simulink model "cpm_jap_r2019a"  (R2019a)
settings: Solver=ode4  StartTime=0.0  StopTime=inf  FixedStep=StepSize  RelTol=1e-3  EnableMultiTasking=on
PostLoadFcn:
  | %% PARAMETER INITIALIZATION
  | modelname = gcs;
  | p = Simulink.Mask.get([modelname, '/CP Model']);
  | 
  | %% HEART
  | % Basal heart period, T0 (s):
  | p.Parameters(1,1).Value = '0.58';
  | %% Right atrium
  | % RA Compliance, Cra (ml/mmHg):
  | p.Parameters(1,2).Value = '31.25';
  | % RA Resistance, Rra (mmHg s/ml):
  | p.Parameters(1,3).Value = '0.0025';
  | % RA Unstressed volume, Vu_ra (ml):
  | p.Parameters(1,4).Value = '22';
  | %% Left atrium
  | % LA Compliance, Cla (ml/mmHg):
  | p.Parameters(1,5).Value = '19.23';
  | % LA Resistance, Rla (mmHg s/ml):
  | p.Parameters(1,6).Value = '0.0025';
  | % LA Unstressed volume, Vu_la (ml):
  | p.Parameters(1,7).Value = '22';
  | %% Right ventricle
  | % RV Resistance coefficient, kR_rv (s/ml):
  | p.Parameters(1,8).Value = '0.0014';
  | % RV free wall End-systolic maximal elastance, Emax_rvf0 (mmHg/ml):
  | p.Parameters(1,9).Value = '1.412';
  | % RV free wall End-systolic unstressed volume, Vu_rvf (ml):
  | p.Parameters(1,10).Value = '35.904';
  | % RV free wall End-diastolic pressure intercept, P0_rvf (mmHg):
  | p.Parameters(1,11).Value = '1.5';
  | % RV free wall End-diastolic elastance coefficient, kE_rvf (1/ml):
  | p.Parameters(1,12).Value = '0.011';
  | % RV free wall Contraction delay (s):
  | p.Parameters(1,13).Value = '0';
  | %% Left ventricle
  | % LV Resistance coefficient, kR_lv (s/ml):
  | p.Parameters(1,14).Value = '0.00037';
  | % LV free wall End-systolic maximal elastance, Emax_lvf0 (mmHg/ml):
  | p.Parameters(1,15).Value = '2.392';
  | % LV free wall End-systolic unstressed volume, Vu_lvf (ml):
  | p.Parameters(1,16).Value = '14.7576';
  | % LV free wall End-diastolic pressure intercept, P0_lvf (mmHg):
  | p.Parameters(1,17).Value = '1.5';
  | % LV free wall End-diastolic elastance coefficient, kE_lvf (1/ml):
  | p.Parameters(1,18).Value = '0.014';
  | % LV Contraction delay (s):
  | p.Parameters(1,19).Value = '0';
  | %% Septum
  | % Septal End-systolic maximal elastance, Emax_spt0 (mmHg/ml):
  | p.Parameters(1,20).Value = '32.4';
  | % Septal End-systolic unstressed volume, Vu_spt (ml):
  | p.Parameters(1,21).Value = '0';
  | % Septal End-diastolic pressure intercept, P0_spt (mmHg):
  | p.Parameters(1,22).Value = '1.11';
  | % Septal End-diastolic elastance coefficient, kE_spt (1/ml):
  | p.Parameters(1,23).Value = '0.175';
  | %% Pericardium
  | % Pericardial Unstressed volume, Vu_pcd (ml):
  | p.Parameters(1,24).Value = '200';
  | % Pericardial Pressure intercept, P0_pcd (mmHg):
  | p.Parameters(1,25).Value = '0.5';
  | % Pericardial Elastance coefficient, kE_pcd (1/ml):
  | p.Parameters(1,26).Value = '0.005';
  | % Pericardial volume, V_pcd (ml):
  | p.Parameters(1,27).Value = '40';
  | 
  | %% LUNGS
  | % Endotracheal tube resistance, Ret (cmH2O/l/s):
  | p.Parameters(1,28).Value = '0';
  | % Lungs resistance, R_L (cmH2O/l/s):
  | p.Parameters(1,29).Value = '1.7459';
  | % Lungs compliance, C_L (l/cmH2O):
  | p.Parameters(1,30).Value = '0.2';
  | % Lungs unstressed volume, Vu_L (l):
  | p.Parameters(1,31).Value = '1.25';
  | % Chest wall compliance, C_cw (l/cmH2O):
  | p.Parameters(1,32).Value = '0.2445';
  | % Chest wall unstressed volume, Vu_cw (l):
  | p.Parameters(1,33).Value = '3.473';
  | % Basal amplitude (cmH2O):
  | p.Parameters(1,34).Value = '5';
  | % Basal frequency (breaths/min):
  | p.Parameters(1,35).Value = '12';
  | % I:E ratio:
  | p.Parameters(1,36).Value = '0.6';
  | % Check for passive patient:
  | p.Parameters(1,37).Value = 'off';
  | % Change in expiratory resistance value (for COPD cases):
  | p.Parameters(1,38).Value = '1';
  | 
  | %% CIRCULATION
  | %% Systemic arteries
  | % Systemic arterial Compliance, Csa (ml/mmHg):
  | p.Parameters(1,39).Value = '0.28';
  | % Systemic arterial Resistance, Rsa (mmHg s/ml):
  | p.Parameters(1,40).Value = '0.06';
  | % Systemic arterial Inertance, Lsa (mmHg ml/s^2):
  | p.Parameters(1,41).Value = '0.00022';
  | % Systemic arterial Unstressed volume, Vu_sa (ml):
  | p.Parameters(1,42).Value = '0';
  | %% Systemic Splanchnic
  | % Systemic Splanchnic peripheral Compliance, Csp (ml/mmHg):
  | p.Parameters(1,43).Value = '2.05';
  | % Systemic Splanchnic peripheral Basal resistance, Rsp_0 (mmHg s/ml):
  | p.Parameters(1,44).Value = '2.49';
  | % Systemic Splanchnic peripheral Unstressed volume, Vu_sp (ml):
  | p.Parameters(1,45).Value = '274.4';
  | % Systemic Splanchnic venous Compliance, Csv (ml/mmHg):
  | p.Parameters(1,46).Value = '42.777';
  | % Systemic Splanchnic venous Resistance, Rsv (mmHg s/ml):
  | p.Parameters(1,47).Value = '0.038';
  | % Systemic Splanchnic venous Basal unstressed volume, Vu_sv_0 (ml):
  | p.Parameters(1,48).Value = '1435.4';
  | %% Systemic Extrasplanchnic
  | % Systemic Extrasplanchnic peripheral Compliance, Cep (ml/mmHg):
  | p.Parameters(1,49).Value = '1.67';
  | % Systemic Extrasplanchnic peripheral Basal resistance, Rep_0 (mmHg s/ml):
  | p.Parameters(1,50).Value = '0.78';
  | % Systemic Extrasplanchnic peripheral Unstressed volume, Vu_ep (ml):
  | p.Parameters(1,51).Value = '336.6';
  | % Systemic Extrasplanchnic venous Compliance, Cev (ml/mmHg):
  | p.Parameters(1,52).Value = '35';
  | % Systemic Extrasplanchnic venous Resistance, Rev (mmHg s/ml):
  | p.Parameters(1,53).Value = '0.016';
  | % Systemic Extrasplanchnic venous Basal unstressed volume, Vu_ev_0 (ml):
  | p.Parameters(1,54).Value = '1537';
  | %% Thoracic veins
  | % Thoracic veins Compliance, Cvc (ml/mmHg):
  | p.Parameters(1,55).Value = '6.6667';
  | % Thoracic veins Basal resistance, Rvc_0 (mmHg s/ml):
  | p.Parameters(1,56).Value = '0.025';
  | % Thoracic veins Unstressed volume, Vu_vc (ml):
  | p.Parameters(1,57).Value = '130';
  | %% Pulmonary arteries
  | % Pulmonary arterial Compliance, Cpa (ml/mmHg):
  | p.Parameters(1,58).Value = '0.76';
  | % Pulmonary arterial Resistance, Rpa (mmHg s/ml):
  | p.Parameters(1,59).Value = '0.023';
  | % Pulmonary arterial Inertance, Lpa (mmHg ml/s^2):
  | p.Parameters(1,60).Value = '0.00018';
  | % Pulmonary arterial Unstressed volume, Vu_pa (ml):
  | p.Parameters(1,61).Value = '0';
  | %% Pulmonary peripheral vessels
  | % Pulmonary peripheral Compliance, Cpp_tot (ml/mmHg):
  | p.Parameters(1,62).Value = '5.80';
  | % Pulmonary peripheral Resistance, Rpp_tot (mmHg s/ml):
  | p.Parameters(1,63).Value = '0.0894';
  | % Pulmonary peripheral Unstressed volume, Vu_pp (ml):
  | p.Parameters(1,64).Value = '108.24';
  | %% Pulmonary veins
  | % Pulmonary venous Compliance, Cpv (ml/mmHg):
  | p.Parameters(1,65).Value = '25.37';
  | % Pulmonary venous Resistance, Rpv (mmHg s/ml):
  | p.Parameters(1,66).Value = '0.0056';
  | % Pulmonary venous Unstressed volume, Vu_pv (ml):
  | p.Parameters(1,67).Value = '105.6';
  | % Basal blood volume, Vt (ml):
  | p.Parameters(1,68).Value = '5300';
  | % Blood infusion Enable?
  | p.Parameters(1,69).Value = 'off';
  | % Blood infusion Duration (min):
  | p.Parameters(1,70).Value = '30';
  | % Blood infusion Volume (ml):
  | p.Parameters(1,71).Value = '500';
  | 
  | %% NEURAL
  | %% Receptors
  | % Baroreceptors set point (mmHg):
  | p.Parameters(1,72).Value = '92';
  | % Baroreceptors Sensitivity (mmHg):
  | p.Parameters(1,73).Value = '11.758';
  | % Central chemoreceptors set point (mmHg):
  | p.Parameters(1,74).Value = '40';
  | % Peripheral chemoreceptors set point (spike/s):
  | p.Parameters(1,75).Value = '3.60';
  | % Central chemoreceptors ampl. sensitivity (dyn/cm^2/mmHg):
  | p.Parameters(1,76).Value = '850';
  | % Perip. chemoreceptors ampl. sensitivity (dyn/cm^2/sp/s):
  | p.Parameters(1,77).Value = '1310';
  | % Central chemoreceptors freq. sensitivity (bpm/mmHg):
  | p.Parameters(1,78).Value = '0.9';
  | % Perip. chemoreceptors freq. sensitivity (bpm/sp/s):
  | p.Parameters(1,79).Value = '0.873474';
  | % Lung-stretch receptors Sensitivity (spkes/l/s)
  | p.Parameters(1,80).Value = '11.76';
  | %% Sympathetic
  | % Baroreceptors's sympathetic influence on heart
  | p.Parameters(1,81).Value = '-1.75';
  | % Peripheral chemoreceptors's sympathetic influence on heart
  | p.Parameters(1,82).Value = '1';
  | % Lung-stretch receptors's sympathetic influence on heart
  | p.Parameters(1,83).Value = '0';
  | % Baroreceptors's sympathetic influence on peripheral circulation
  | p.Parameters(1,84).Value = '-1.1375';
  | % Peripheral chemoreceptors's sympathetic influence on peripheral circulation
  | p.Parameters(1,85).Value = '1.716';
  | % Lung-stretch receptors's sympathetic influence on peripheral circulation
  | p.Parameters(1,86).Value = '-0.3997';
  | % Baroreceptors's sympathetic influence on venous circulation
  | p.Parameters(1,87).Value = '-1.0806';
  | % Peripheral chemoreceptors's sympathetic influence on venous circulation
  | p.Parameters(1,88).Value = '1.716';
  | % Lung-stretch receptors's sympathetic influence on venous circulation
  | p.Parameters(1,89).Value = '-0.2907';
  | %% Vagal
  | % Baroreceptors's vagal influence on heart
  | p.Parameters(1,90).Value = '7.06';
  | % Peripheral chemoreceptors's vagal influence on peripheral circulation
  | p.Parameters(1,91).Value = '0.208';
  | % Peripheral chemoreceptors's vagal influence on venous circulation
  | p.Parameters(1,92).Value = '-0.103';
  | %% CNS Ischemic response
  | % PO2 sensitivity heart (mmHg):
  | p.Parameters(1,93).Value = '45';
  | % PO2 sensitivity peripheral circulation (mmHg):
  | p.Parameters(1,94).Value = '30';
  | % PO2 sensitivity venous circulation (mmHg):
  | p.Parameters(1,95).Value = '30';
  | % PCO2 sensitivity heart (1/(mmHg s)):
  | p.Parameters(1,96).Value = '1';
  | % PCO2 sensitivity peripheral circulation (1/(mmHg s)):
  | p.Parameters(1,97).Value = '1.5';
  | % PCO2 sensitivity Veins (1/(mmHg s)):
  | p.Parameters(1,98).Value = '0';
  | 
  | %% METABOLISM
  | % Splanchnic Oxygen consumption (ml/min):
  | p.Parameters(1,99).Value = '108.419';
  | % Splanchnic Carbon dioxide production (ml/min):
  | p.Parameters(1,100).Value = '91.072';
  | % Splanchnic Tissue volume (ml):
  | p.Parameters(1,101).Value = '2673';
  | % Extrasplanchnic Oxygen consumption (ml/min):
  | p.Parameters(1,102).Value = '137.785';
  | % Extrasplanchnic Carbon dioxide production (ml/min):
  | p.Parameters(1,103).Value = '115.7394';
  | % Extrasplanchnic Tissue volume (ml):
  | p.Parameters(1,104).Value = '33046';
  | 
  | %% GAS EXCHANGE
  | % Oxygen air fraction, FiO2 (%):
  | p.Parameters(1,105).Value = '21.0379';
  | % Carbon dioxide air fraction, FiCO2 (%):
  | p.Parameters(1,106).Value = '0.042076';
  | % Pulmonary shunt, sh (%):
  | p.Parameters(1,107).Value = '1.7';
  | % Deadspace volume, Vdead (l):
  | p.Parameters(1,108).Value = '0.15';
InitFcn:
  | logFreq = 100; % logging frequency
  | StepSize = 5e-4; % simulation step size
  | 
  | %% PARAMETER INITIALIZATION
  | modelname = gcs;
  | p = Simulink.Mask.get([modelname, '/CP Model']);
  | 
  | %% HEART
  | % Basal heart period, T0 (s):
  | p.Parameters(1,1).Value = '0.58';
  | %% Right atrium
  | % RA Compliance, Cra (ml/mmHg):
  | p.Parameters(1,2).Value = '31.25';
  | % RA Resistance, Rra (mmHg s/ml):
  | p.Parameters(1,3).Value = '0.0025';
  | % RA Unstressed volume, Vu_ra (ml):
  | p.Parameters(1,4).Value = '22';
  | %% Left atrium
  | % LA Compliance, Cla (ml/mmHg):
  | p.Parameters(1,5).Value = '19.23';
  | % LA Resistance, Rla (mmHg s/ml):
  | p.Parameters(1,6).Value = '0.0025';
  | % LA Unstressed volume, Vu_la (ml):
  | p.Parameters(1,7).Value = '22';
  | %% Right ventricle
  | % RV Resistance coefficient, kR_rv (s/ml):
  | p.Parameters(1,8).Value = '0.0014';
  | % RV free wall End-systolic maximal elastance, Emax_rvf0 (mmHg/ml):
  | p.Parameters(1,9).Value = '1.412';
  | % RV free wall End-systolic unstressed volume, Vu_rvf (ml):
  | p.Parameters(1,10).Value = '35.904';
  | % RV free wall End-diastolic pressure intercept, P0_rvf (mmHg):
  | p.Parameters(1,11).Value = '1.5';
  | % RV free wall End-diastolic elastance coefficient, kE_rvf (1/ml):
  | p.Parameters(1,12).Value = '0.011';
  | % RV free wall Contraction delay (s):
  | p.Parameters(1,13).Value = '0';
  | %% Left ventricle
  | % LV Resistance coefficient, kR_lv (s/ml):
  | p.Parameters(1,14).Value = '0.00037';
  | % LV free wall End-systolic maximal elastance, Emax_lvf0 (mmHg/ml):
  | p.Parameters(1,15).Value = '2.392';
  | % LV free wall End-systolic unstressed volume, Vu_lvf (ml):
  | p.Parameters(1,16).Value = '14.7576';
  | % LV free wall End-diastolic pressure intercept, P0_lvf (mmHg):
  | p.Parameters(1,17).Value = '1.5';
  | % LV free wall End-diastolic elastance coefficient, kE_lvf (1/ml):
  | p.Parameters(1,18).Value = '0.014';
  | % LV Contraction delay (s):
  | p.Parameters(1,19).Value = '0';
  | %% Septum
  | % Septal End-systolic maximal elastance, Emax_spt0 (mmHg/ml):
  | p.Parameters(1,20).Value = '32.4';
  | % Septal End-systolic unstressed volume, Vu_spt (ml):
  | p.Parameters(1,21).Value = '0';
  | % Septal End-diastolic pressure intercept, P0_spt (mmHg):
  | p.Parameters(1,22).Value = '1.11';
  | % Septal End-diastolic elastance coefficient, kE_spt (1/ml):
  | p.Parameters(1,23).Value = '0.175';
  | %% Pericardium
  | % Pericardial Unstressed volume, Vu_pcd (ml):
  | p.Parameters(1,24).Value = '200';
  | % Pericardial Pressure intercept, P0_pcd (mmHg):
  | p.Parameters(1,25).Value = '0.5';
  | % Pericardial Elastance coefficient, kE_pcd (1/ml):
  | p.Parameters(1,26).Value = '0.005';
  | % Pericardial volume, V_pcd (ml):
  | p.Parameters(1,27).Value = '40';
  | 
  | %% LUNGS
  | % Endotracheal tube resistance, Ret (cmH2O/l/s):
  | p.Parameters(1,28).Value = '0';
  | % Lungs resistance, R_L (cmH2O/l/s):
  | p.Parameters(1,29).Value = '1.7459';
  | % Lungs compliance, C_L (l/cmH2O):
  | p.Parameters(1,30).Value = '0.2';
  | % Lungs unstressed volume, Vu_L (l):
  | p.Parameters(1,31).Value = '1.25';
  | % Chest wall compliance, C_cw (l/cmH2O):
  | p.Parameters(1,32).Value = '0.2445';
  | % Chest wall unstressed volume, Vu_cw (l):
  | p.Parameters(1,33).Value = '3.473';
  | % Basal amplitude (cmH2O):
  | p.Parameters(1,34).Value = '5';
  | % Basal frequency (breaths/min):
  | p.Parameters(1,35).Value = '12';
  | % I:E ratio:
  | p.Parameters(1,36).Value = '0.6';
  | % Check for passive patient:
  | p.Parameters(1,37).Value = 'off';
  | % Change in expiratory resistance value (for COPD cases):
  | p.Parameters(1,38).Value = '1';
  | 
  | %% CIRCULATION
  | %% Systemic arteries
  | % Systemic arterial Compliance, Csa (ml/mmHg):
  | p.Parameters(1,39).Value = '0.28';
  | % Systemic arterial Resistance, Rsa (mmHg s/ml):
  | p.Parameters(1,40).Value = '0.06';
  | % Systemic arterial Inertance, Lsa (mmHg ml/s^2):
  | p.Parameters(1,41).Value = '0.00022';
  | % Systemic arterial Unstressed volume, Vu_sa (ml):
  | p.Parameters(1,42).Value = '0';
  | %% Systemic Splanchnic
  | % Systemic Splanchnic peripheral Compliance, Csp (ml/mmHg):
  | p.Parameters(1,43).Value = '2.05';
  | % Systemic Splanchnic peripheral Basal resistance, Rsp_0 (mmHg s/ml):
  | p.Parameters(1,44).Value = '2.49';
  | % Systemic Splanchnic peripheral Unstressed volume, Vu_sp (ml):
  | p.Parameters(1,45).Value = '274.4';
  | % Systemic Splanchnic venous Compliance, Csv (ml/mmHg):
  | p.Parameters(1,46).Value = '42.777';
  | % Systemic Splanchnic venous Resistance, Rsv (mmHg s/ml):
  | p.Parameters(1,47).Value = '0.038';
  | % Systemic Splanchnic venous Basal unstressed volume, Vu_sv_0 (ml):
  | p.Parameters(1,48).Value = '1435.4';
  | %% Systemic Extrasplanchnic
  | % Systemic Extrasplanchnic peripheral Compliance, Cep (ml/mmHg):
  | p.Parameters(1,49).Value = '1.67';
  | % Systemic Extrasplanchnic peripheral Basal resistance, Rep_0 (mmHg s/ml):
  | p.Parameters(1,50).Value = '0.78';
  | % Systemic Extrasplanchnic peripheral Unstressed volume, Vu_ep (ml):
  | p.Parameters(1,51).Value = '336.6';
  | % Systemic Extrasplanchnic venous Compliance, Cev (ml/mmHg):
  | p.Parameters(1,52).Value = '35';
  | % Systemic Extrasplanchnic venous Resistance, Rev (mmHg s/ml):
  | p.Parameters(1,53).Value = '0.016';
  | % Systemic Extrasplanchnic venous Basal unstressed volume, Vu_ev_0 (ml):
  | p.Parameters(1,54).Value = '1537';
  | %% Thoracic veins
  | % Thoracic veins Compliance, Cvc (ml/mmHg):
  | p.Parameters(1,55).Value = '6.6667';
  | % Thoracic veins Basal resistance, Rvc_0 (mmHg s/ml):
  | p.Parameters(1,56).Value = '0.025';
  | % Thoracic veins Unstressed volume, Vu_vc (ml):
  | p.Parameters(1,57).Value = '130';
  | %% Pulmonary arteries
  | % Pulmonary arterial Compliance, Cpa (ml/mmHg):
  | p.Parameters(1,58).Value = '0.76';
  | % Pulmonary arterial Resistance, Rpa (mmHg s/ml):
  | p.Parameters(1,59).Value = '0.023';
  | % Pulmonary arterial Inertance, Lpa (mmHg ml/s^2):
  | p.Parameters(1,60).Value = '0.00018';
  | % Pulmonary arterial Unstressed volume, Vu_pa (ml):
  | p.Parameters(1,61).Value = '0';
  | %% Pulmonary peripheral vessels
  | % Pulmonary peripheral Compliance, Cpp_tot (ml/mmHg):
  | p.Parameters(1,62).Value = '5.80';
  | % Pulmonary peripheral Resistance, Rpp_tot (mmHg s/ml):
  | p.Parameters(1,63).Value = '0.0894';
  | % Pulmonary peripheral Unstressed volume, Vu_pp (ml):
  | p.Parameters(1,64).Value = '108.24';
  | %% Pulmonary veins
  | % Pulmonary venous Compliance, Cpv (ml/mmHg):
  | p.Parameters(1,65).Value = '25.37';
  | % Pulmonary venous Resistance, Rpv (mmHg s/ml):
  | p.Parameters(1,66).Value = '0.0056';
  | % Pulmonary venous Unstressed volume, Vu_pv (ml):
  | p.Parameters(1,67).Value = '105.6';
  | % Basal blood volume, Vt (ml):
  | p.Parameters(1,68).Value = '5300';
  | % Blood infusion Enable?
  | p.Parameters(1,69).Value = 'off';
  | % Blood infusion Duration (min):
  | p.Parameters(1,70).Value = '30';
  | % Blood infusion Volume (ml):
  | p.Parameters(1,71).Value = '500';
  | 
  | %% NEURAL
  | %% Receptors
  | % Baroreceptors set point (mmHg):
  | p.Parameters(1,72).Value = '92';
  | % Baroreceptors Sensitivity (mmHg):
  | p.Parameters(1,73).Value = '11.758';
  | % Central chemoreceptors set point (mmHg):
  | p.Parameters(1,74).Value = '40';
  | % Peripheral chemoreceptors set point (spike/s):
  | p.Parameters(1,75).Value = '3.60';
  | % Central chemoreceptors ampl. sensitivity (dyn/cm^2/mmHg):
  | p.Parameters(1,76).Value = '850';
  | % Perip. chemoreceptors ampl. sensitivity (dyn/cm^2/sp/s):
  | p.Parameters(1,77).Value = '1310';
  | % Central chemoreceptors freq. sensitivity (bpm/mmHg):
  | p.Parameters(1,78).Value = '0.9';
  | % Perip. chemoreceptors freq. sensitivity (bpm/sp/s):
  | p.Parameters(1,79).Value = '0.873474';
  | % Lung-stretch receptors Sensitivity (spkes/l/s)
  | p.Parameters(1,80).Value = '11.76';
  | %% Sympathetic
  | % Baroreceptors's sympathetic influence on heart
  | p.Parameters(1,81).Value = '-1.75';
  | % Peripheral chemoreceptors's sympathetic influence on heart
  | p.Parameters(1,82).Value = '1';
  | % Lung-stretch receptors's sympathetic influence on heart
  | p.Parameters(1,83).Value = '0';
  | % Baroreceptors's sympathetic influence on peripheral circulation
  | p.Parameters(1,84).Value = '-1.1375';
  | % Peripheral chemoreceptors's sympathetic influence on peripheral circulation
  | p.Parameters(1,85).Value = '1.716';
  | % Lung-stretch receptors's sympathetic influence on peripheral circulation
  | p.Parameters(1,86).Value = '-0.3997';
  | % Baroreceptors's sympathetic influence on venous circulation
  | p.Parameters(1,87).Value = '-1.0806';
  | % Peripheral chemoreceptors's sympathetic influence on venous circulation
  | p.Parameters(1,88).Value = '1.716';
  | % Lung-stretch receptors's sympathetic influence on venous circulation
  | p.Parameters(1,89).Value = '-0.2907';
  | %% Vagal
  | % Baroreceptors's vagal influence on heart
  | p.Parameters(1,90).Value = '7.06';
  | % Peripheral chemoreceptors's vagal influence on peripheral circulation
  | p.Parameters(1,91).Value = '0.208';
  | % Peripheral chemoreceptors's vagal influence on venous circulation
  | p.Parameters(1,92).Value = '-0.103';
  | %% CNS Ischemic response
  | % PO2 sensitivity heart (mmHg):
  | p.Parameters(1,93).Value = '45';
  | % PO2 sensitivity peripheral circulation (mmHg):
  | p.Parameters(1,94).Value = '30';
  | % PO2 sensitivity venous circulation (mmHg):
  | p.Parameters(1,95).Value = '30';
  | % PCO2 sensitivity heart (1/(mmHg s)):
  | p.Parameters(1,96).Value = '1';
  | % PCO2 sensitivity peripheral circulation (1/(mmHg s)):
  | p.Parameters(1,97).Value = '1.5';
  | % PCO2 sensitivity Veins (1/(mmHg s)):
  | p.Parameters(1,98).Value = '0';
  | 
  | %% METABOLISM
  | % Splanchnic Oxygen consumption (ml/min):
  | p.Parameters(1,99).Value = '108.419';
  | % Splanchnic Carbon dioxide production (ml/min):
  | p.Parameters(1,100).Value = '91.072';
  | % Splanchnic Tissue volume (ml):
  | p.Parameters(1,101).Value = '2673';
  | % Extrasplanchnic Oxygen consumption (ml/min):
  | p.Parameters(1,102).Value = '137.785';
  | % Extrasplanchnic Carbon dioxide production (ml/min):
  | p.Parameters(1,103).Value = '115.7394';
  | % Extrasplanchnic Tissue volume (ml):
  | p.Parameters(1,104).Value = '33046';
  | 
  | %% GAS EXCHANGE
  | % Oxygen air fraction, FiO2 (%):
  | p.Parameters(1,105).Value = '21.0379';
  | % Carbon dioxide air fraction, FiCO2 (%):
  | p.Parameters(1,106).Value = '0.042076';
  | % Pulmonary shunt, sh (%):
  | p.Parameters(1,107).Value = '1.7';
  | % Deadspace volume, Vdead (l):
  | p.Parameters(1,108).Value = '0.15';
StopFcn:
  | cpmResults = cpm_jap{1}.Values;
(part 1 of 2)
settings Model: ParamWorkspaceSource=ReferencedWorkspace  TunableVars=BreathAmp,BreathFreq,CL,C_cw,C_vc,Cep,Cev,Cla,ConsCO2Exspl,ConsCO2Spl,ConsO2Exspl,ConsO2Spl,Cpa,Cpp_tot,Cpv,Cra,Csa,Csp,Csv,Ees_spt0,Emax_lvf0,Emax_rvf0,ExsplVolume,FRCnom,FiCO2,FiO2,Gc_A_up,Gc_f_up,Gp_A_up,Gp_f_up,Gsr,IEratio,Lpa,Lsa,P0_lvf,P0_pcd,P0_rvf,P0_spt,PO2sh,PO2sp,PO2sv,PaCO2n,Pn,RL,R_vc_0,Rep_0,Ret,Rev,Rla,Rpa,Rpp_tot,Rpv,Rra,Rsa,Rsp_0,Rsv,SplVolume,T0,V0_pcd,V0_spt,V_pcd,Vdead,Vt,Vu_L,Vu_cw,Vu_ep,Vu_ev0,Vu_la,Vu_lvf,Vu_pa,Vu_pp,Vu_ps,Vu_pv,Vu_ra,Vu_rvf,Vu_sa,Vu_sp,Vu_sv0,Vu_vc,Wbsh,Wbsp,Wbsv,Wpcsh,Wpcsp,Wpcsv,Wpcv,Wsrsh,Wsrsp,Wsrsv,Wsrv,fapcn,gccsh,gccsp,gccsv,infusionDur,kBloodLoss,kE_lvf,kE_rvf,kRL_out,kR_lv,kR_rv,kab,kev,lambda_pcd,lambda_spt,lvContractionDelay,passivePatient,pumpFlag,rvContractionDelay,sh,volumeInfused  TunableVarsStorageClass=Auto,Auto,Auto,Auto,Auto,Auto,Auto,Auto,Auto,Auto,Auto,Auto,Auto,Auto,Auto,Auto,Auto,Auto,Auto,Auto,Auto,Auto,Auto,Auto,Auto,Auto,Auto,Auto,Auto,Auto,Auto,Auto,Auto,Auto,Auto,Auto,Auto,Auto,Auto,Auto,Auto,Auto,Auto,Auto,Auto,Auto,Auto,Auto,Auto,Auto,Auto,Auto,Auto,Auto,Auto,Auto,Auto,Auto,Auto,Auto,Auto,Auto,Auto,Auto,Auto,Auto,Auto,Auto,Auto,Auto,Auto,Auto,Auto,Auto,Auto,Auto,Auto,Auto,Auto,Auto,Auto,Auto,Auto,Auto,Auto,Auto,Auto,Auto,Auto,Auto,Auto,Auto,Auto,Auto,Auto,Auto,Auto,Auto,Auto,Auto,Auto,Auto,Auto,Auto,Auto,Auto,Auto,Auto,Auto,Auto,Auto  TunableVarsTypeQualifier=,,,,,,,,,,,,,,,,,,,,,,,,,,,,,,,,,,,,,,,,,,,,,,,,,,,,,,,,,,,,,,,,,,,,,,,,,,,,,,,,,,,,,,,,,,,,,,,,,,,,,,,,,,,,,,  Creator=nikolaos  LastModifiedBy=nikolaos
settings DataIOCC: SaveOutput=off  SaveTime=off  ReturnWorkspaceOutputs=off  SignalLoggingName=cpm_jap
settings OptimizationCC: BlockReduction=off  DefaultParameterBehavior=Inlined  OptimizeBlockIOStorage=off  BufferReuse=off  GlobalBufferReuse=off  ExpressionFolding=off  LocalBlockOutputs=off  OptimizeDataStoreBuffers=off  BusAssignmentInplaceUpdate=off
settings DebuggingCC: UnderspecifiedInitializationDetection=Classic  MergeDetectMultiDrivingBlocksExec=none  PregeneratedLibrarySubsystemCodeDiagnostic=none  ArithmeticOperatorsInVariantConditions=warning
settings SFSimCC: SimUseLocalCustomCode=off
settings RTWCC: RTWUseLocalCustomCode=off
settings ConfigComp: CovMetricSettings=dw  CovHtmlReporting=on  CovSaveCumulativeToWorkspaceVar=on  CovSaveSingleToWorkspaceVar=on  CovExternalEMLEnable=off

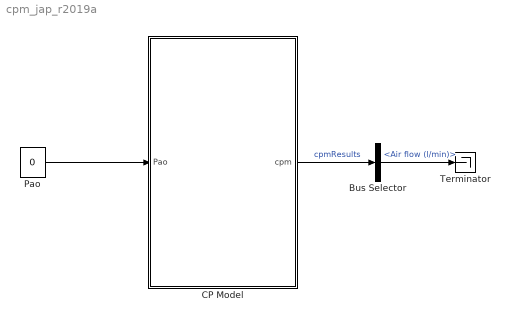
== system cpm_jap_r2019a ==
  Bus Selector : BusSelector  OutputSignals=lungs.Air flow (l/min)
  CP Model : Subsystem  mask(CP Model){sfcnParam58=0.58, sfcnParam16=31.25, sfcnParam53=0.0025, sfcnParam74=22, sfcnParam8=19.23, sfcnParam49=0.0025, sfcnParam68=22, sfcnParam101=0.0014, sfcnParam22=1.412, sfcnParam75=35.904, sfcnParam37=1.5, sfcnParam98=0.011, sfcnParam109=0, sfcnParam100=0.00037, sfcnParam21=2.392, sfcnParam69=14.7576, sfcnParam35=1.5, sfcnParam97=0.014, sfcnParam106=0, sfcnParam20=32.4, sfcnParam60=0, sfcnParam38=1.11, sfcnParam105=0.175, sfcnParam59=200, sfcnParam36=0.5, sfcnParam104=0.005, sfcnParam61=40, sfcnParam47=0, sfcnParam44=1.7459, sfcnParam3=0.2, sfcnParam64=1.25, sfcnParam4=0.2445, sfcnParam65=3.473, sfcnParam1=5, sfcnParam2=12, sfcnParam32=0.6, sfcnParam107=off, sfcnParam99=1, sfcnParam17=0.28, sfcnParam54=0.06, sfcnParam34=0.00022, sfcnParam76=0, sfcnParam18=2.05, sfcnParam55=2.49, sfcnParam77=274.4, sfcnParam19=42.777, sfcnParam56=0.038, sfcnParam78=1435.4, sfcnParam6=1.67, sfcnParam46=0.78, sfcnParam66=336.6, sfcnParam7=35, sfcnParam48=0.016, sfcnParam67=1537, sfcnParam5=6.6667, sfcnParam45=0.025, sfcnParam79=130, sfcnParam13=0.76, sfcnParam50=0.023, sfcnParam33=0.00018, sfcnParam70=0, sfcnParam14=5.80, sfcnParam51=0.0894, sfcnParam71=108.24, sfcnParam15=25.37, sfcnParam52=0.0056, sfcnParam73=105.6, sfcnParam63=5300, sfcnParam108=off, sfcnParam95=30, sfcnParam111=500, sfcnParam43=92, sfcnParam102=11.758, sfcnParam42=40, sfcnParam91=3.60, sfcnParam27=850, sfcnParam29=1310, sfcnParam28=0.9, sfcnParam30=0.873474, sfcnParam31=11.76, sfcnParam80=-1.75, sfcnParam83=1, sfcnParam87=0, sfcnParam81=-1.1375, sfcnParam84=1.716, sfcnParam88=-0.3997, sfcnParam82=-1.0806, sfcnParam85=1.716, sfcnParam89=-0.2907, sfcnParam103=7.06, sfcnParam86=0.208, sfcnParam90=-0.103, sfcnParam39=45, sfcnParam40=30, sfcnParam41=30, sfcnParam92=1, sfcnParam93=1.5, sfcnParam94=0, sfcnParam12=108.419, sfcnParam10=91.072, sfcnParam57=2673, sfcnParam11=137.785, sfcnParam9=115.7394, sfcnParam23=33046, sfcnParam26=21.0379, sfcnParam25=0.042076, sfcnParam110=1.7, sfcnParam62=0.15}
      mask prompts: sfcnParam58 "Basal heart period, T0 (s):"; sfcnParam16 "Compliance, Cra (ml/mmHg):"; sfcnParam53 "Resistance, Rra (mmHg s/ml):"; sfcnParam74 "Unstressed volume, Vu_ra (ml):"; sfcnParam8 "Compliance, Cla (ml/mmHg):"; sfcnParam49 "Resistance, Rla (mmHg s/ml):"; sfcnParam68 "Unstressed volume, Vu_la (ml):"; sfcnParam101 "Resistance coefficient, kR_rv (s/ml):"; sfcnParam22 "End-systolic maximal elastance, Emax_rvf0 (mmHg/ml):"; sfcnParam75 "End-systolic unstressed volume, Vu_rvf (ml):"; sfcnParam37 "End-diastolic pressure intercept, P0_rvf (mmHg):"; sfcnParam98 "End-diastolic elastance coefficient, kE_rvf (1/ml):"; sfcnParam109 "Contraction delay (s):"; sfcnParam100 "Resistance coefficient, kR_lv (s/ml):"; sfcnParam21 "End-systolic maximal elastance, Emax_lvf0 (mmHg/ml):"; sfcnParam69 "End-systolic unstressed volume, Vu_lvf (ml):"; sfcnParam35 "End-diastolic pressure intercept, P0_lvf (mmHg):"; sfcnParam97 "End-diastolic elastance coefficient, kE_lvf (1/ml):"; sfcnParam106 "Contraction delay (s):"; sfcnParam20 "End-systolic maximal elastance, Emax_spt0 (mmHg/ml):"; sfcnParam60 "End-systolic unstressed volume, Vu_spt (ml):"; sfcnParam38 "End-diastolic pressure intercept, P0_spt (mmHg):"; sfcnParam105 "End-diastolic elastance coefficient, kE_spt (1/ml):"; sfcnParam59 "Unstressed volume, Vu_pcd (ml):"; sfcnParam36 "Pressure intercept, P0_pcd (mmHg):"; sfcnParam104 "Elastance coefficient, kE_pcd (1/ml):"; sfcnParam61 "Pericardial volume, V_pcd (ml):"; sfcnParam47 "Endotracheal tube resistance, Ret (cmH2O/l/s):"; sfcnParam44 "Lungs resistance, R_L (cmH2O/l/s):"; sfcnParam3 "Lungs compliance, C_L (l/cmH2O):"; sfcnParam64 "Lungs unstressed volume, Vu_L (l):"; sfcnParam4 "Chest wall compliance, C_cw (l/cmH2O):"; sfcnParam65 "Chest wall unstressed volume, Vu_cw (l):"; sfcnParam1 "Basal amplitude (cmH2O):"; sfcnParam2 "Basal frequency (breaths/min):"; sfcnParam32 "I:E ratio:"; sfcnParam107 "Check for passive patient:"; sfcnParam99 "Change in expiratory resistance value (for COPD cases):"; sfcnParam17 "Compliance, Csa (ml/mmHg):"; sfcnParam54 "Resistance, Rsa (mmHg s/ml):"; sfcnParam34 "Inertance, Lsa (mmHg ml/s^2):"; sfcnParam76 "Unstressed volume, Vu_sa (ml):"; sfcnParam18 "Compliance, Csp (ml/mmHg):"; sfcnParam55 "Basal resistance, Rsp_0 (mmHg s/ml):"; sfcnParam77 "Unstressed volume, Vu_sp (ml):"; sfcnParam19 "Compliance, Csv (ml/mmHg):"; sfcnParam56 "Resistance, Rsv (mmHg s/ml):"; sfcnParam78 "Basal unstressed volume, Vu_sv_0 (ml):"; sfcnParam6 "Compliance, Cep (ml/mmHg):"; sfcnParam46 "Basal resistance, Rep_0 (mmHg s/ml):"; sfcnParam66 "Unstressed volume, Vu_ep (ml):"; sfcnParam7 "Compliance, Cev (ml/mmHg):"; sfcnParam48 "Resistance, Rev (mmHg s/ml):"; sfcnParam67 "Basal unstressed volume, Vu_ev_0 (ml):"; sfcnParam5 "Compliance, Cvc (ml/mmHg):"; sfcnParam45 "Basal resistance, Rvc_0 (mmHg s/ml):"; sfcnParam79 "Unstressed volume, Vu_vc (ml):"; sfcnParam13 "Compliance, Cpa (ml/mmHg):"; sfcnParam50 "Resistance, Rpa (mmHg s/ml):"; sfcnParam33 "Inertance, Lpa (mmHg ml/s^2):"; sfcnParam70 "Unstressed volume, Vu_pa (ml):"; sfcnParam14 "Compliance, Cpp_tot (ml/mmHg):"; sfcnParam51 "Resistance, Rpp_tot (mmHg s/ml):"; sfcnParam71 "Unstressed volume, Vu_pp (ml):"; sfcnParam15 "Compliance, Cpv (ml/mmHg):"; sfcnParam52 "Resistance, Rpv (mmHg s/ml):"; sfcnParam73 "Unstressed volume, Vu_pv (ml):"; sfcnParam63 "Basal blood volume, Vt (ml):"; sfcnParam108 "Enable?"; sfcnParam95 "Duration (min):"; sfcnParam111 "Volume (ml)"; sfcnParam43 "Set point (mmHg):"; sfcnParam102 "Sensitivity (mmHg):"; sfcnParam42 "Central set point (mmHg):"; sfcnParam91 "Peripheral set point (spike/s):"; sfcnParam27 "Central ampl. sensitivity (dyn/cm^2/mmHg):"; sfcnParam29 "Perip. ampl. sensitivity (dyn/cm^2/sp/s):"; sfcnParam28 "Central freq. sensitivity (bpm/mmHg):"; sfcnParam30 "Perip. freq. sensitivity (bpm/sp/s):"; sfcnParam31 "Sensitivity (spkes/l/s)"; sfcnParam80 "Baroreceptors:"; sfcnParam83 "Peripheral chemoreceptors:"; sfcnParam87 "Lung-stretch receptors:"; sfcnParam81 "Baroreceptors:"; sfcnParam84 "Peripheral chemoreceptors:"; sfcnParam88 "Lung-stretch receptors:"; sfcnParam82 "Baroreceptors:"; sfcnParam85 "Peripheral chemoreceptors:"; sfcnParam89 "Lung-stretch receptors:"; sfcnParam103 "Baroreceptors:"; sfcnParam86 "Peripheral chemoreceptors:"; sfcnParam90 "Lung-stretch receptors:"; sfcnParam39 "Heart (mmHg):"; sfcnParam40 "Peripheral circulation (mmHg):"; sfcnParam41 "Veins (mmHg):"; sfcnParam92 "Heart (1/(mmHg s)):"; sfcnParam93 "Peripheral circulation (1/(mmHg s)):"; sfcnParam94 "Veins (1/(mmHg s)):"; sfcnParam12 "Oxygen consumption (ml/min):"; sfcnParam10 "Carbon dioxide production (ml/min):"; sfcnParam57 "Tissue volume (ml):"; sfcnParam11 "Oxygen consumption (ml/min):"; sfcnParam9 "Carbon dioxide production (ml/min):"; sfcnParam23 "Tissue volume (ml):"; sfcnParam26 "Oxygen air fraction, FiO2 (%):"; sfcnParam25 "Carbon dioxide air fraction, FiCO2 (%):"; sfcnParam110 "Pulmonary shunt, sh (%):"; sfcnParam62 "Deadspace volume, Vdead (l):"
      mask help:
      | Heart-lung interactions during mechanical ventilation: Analysis via a cardiopulmonary simulation model
      |
      | Nikolaos Karamolegkos, Antonio Albanese, and Nicolas W. Chbat
      |
      | Journal of Applied Physiology
      |
      | 2019
      mask DialogControl Container4 Prompt: Heart
      mask DialogControl Container5 Prompt: Right atrium
      mask DialogControl Container7 Prompt: Left atrium
      mask DialogControl Container8 Prompt: RV free wall
      mask DialogControl Container9 Prompt: LV free wall
      mask DialogControl Container10 Prompt: Septum
      mask DialogControl Container11 Prompt: Pericardium
      mask DialogControl Container13 Prompt: Lungs
      mask DialogControl Breathing Prompt: Breathing properties
      mask DialogControl sfcnParam99 Tooltip: Value indicates the change in resistance during expiration, e.g., 1.1 is 10% increase in airway resistance.
      mask DialogControl Container18 Prompt: Circulation
      mask DialogControl Container21 Prompt: Systemic
      mask DialogControl Container20 Prompt: Arteries
      mask DialogControl Container23 Prompt: Splanchnic
      mask DialogControl Container24 Prompt: Peripheral
      mask DialogControl Container25 Prompt: Venous
      mask DialogControl Container29 Prompt: Extrasplanchnic
      mask DialogControl Container30 Prompt: Peripheral
      mask DialogControl Container31 Prompt: Venous
      mask DialogControl Container32 Prompt: Thoracic veins
      mask DialogControl Container33 Prompt: Pulmonary
      mask DialogControl Container35 Prompt: Arteries
      mask DialogControl Container36 Prompt: Peripheral (total)
      mask DialogControl Container37 Prompt: Veins
      mask DialogControl Container57 Prompt: Blood infusion
      mask DialogControl sfcnParam108 Tooltip: For every check and uncheck, the selected volume will be administered.
      mask DialogControl Container38 Prompt: Neural
      mask DialogControl Container40 Prompt: Receptors
      mask DialogControl Container41 Prompt: Baroreceptors
      mask DialogControl Container42 Prompt: Chemoreceptors
      mask DialogControl Container43 Prompt: Lung-stretch receptors
      mask DialogControl Container44 Prompt: Sympathetic
      mask DialogControl Container45 Prompt: Receptor's influence on heart
      mask DialogControl Container46 Prompt: Receptor's influence on peripheral circulation
      mask DialogControl Container47 Prompt: Receptor's influence on venous circulation
      mask DialogControl Container48 Prompt: Vagal
      mask DialogControl Container49 Prompt: Receptor's influence on heart
      mask DialogControl Container50 Prompt: CNS Ischemic
      mask DialogControl Container51 Prompt: PO2 sensitivity
      mask DialogControl Container52 Prompt: PCO2 sensitivity
      mask DialogControl Container53 Prompt: Metabolism
      mask DialogControl Container54 Prompt: Splanchnic
      mask DialogControl Container55 Prompt: Extrasplanchnic
      mask DialogControl Container56 Prompt: Gas exchange
  Pao : Constant  Value=0
  Terminator : Terminator
  wires:
  Pao/1 -> CP Model/1(Pao)
  Bus Selector/1 -> Terminator/1  "<Air flow (l/min)>"
  CP Model/1(cpm) -> Bus Selector/1  "cpmResults"
